simulink model "PI_model"  (Simulink 8.1)
settings: Solver=ode3  StartTime=0.0  StopTime=5500  FixedStep=1  RelTol=1e-3
undefined symbols (not defined in the file or in its folder): sys
libraries: simulink x2
settings Model: Creator=Lenovo  LastModifiedBy=Lenovo
settings DebuggingCC: FcnCallInpInsideContextMsg=EnableAllAsWarning

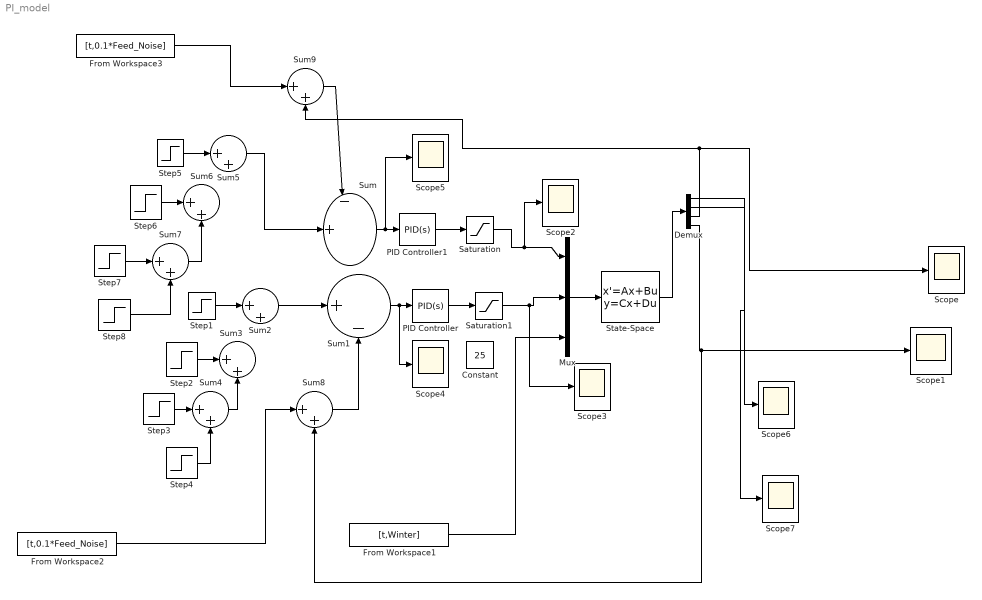
== system PI_model ==
  Constant : Constant  Value=25
  Demux : Demux
  From Workspace1 : FromWorkspace  VariableName=[t,Winter]  SampleTime=0
  From Workspace2 : FromWorkspace  VariableName=[t,0.1*Feed_Noise]  SampleTime=0
  From Workspace3 : FromWorkspace  VariableName=[t,0.1*Feed_Noise]  SampleTime=0
  Mux : Mux  Inputs=3
  PID Controller : simulink/Continuous/PID Controller  Controller=PID  TimeDomain=Continuous-time  SampleTime=1  IntegratorMethod=Forward Euler  FilterMethod=Forward Euler  Form=Parallel  P=8.594*0.5  I=0.17188*2  D=0  N=100  InitialConditionSource=internal  InitialConditionForIntegrator=0  InitialConditionForFilter=0  ExternalReset=none  LimitOutput=off  UpperSaturationLimit=inf  LowerSaturationLimit=-inf  LinearizeAsGain=off  AntiWindupMode=none  Kb=1  TrackingMode=off  Kt=1  PParamMin=[]  PParamMax=[]  IParamMin=[]  IParamMax=[]  DParamMin=[]  DParamMax=[]  NParamMin=[]  NParamMax=[]  KbParamMin=[]  KbParamMax=[]  KtParamMin=[]  KtParamMax=[]  POutMin=[]  POutMax=[]  IOutMin=[]  IOutMax=[]  DOutMin=[]  DOutMax=[]  NOutMin=[]  NOutMax=[]  KbOutMin=[]  KbOutMax=[]  KtOutMin=[]  KtOutMax=[]  IntegratorOutMin=[]  IntegratorOutMax=[]  FilterOutMin=[]  FilterOutMax=[]  SumOutMin=[]  SumOutMax=[]  SumI1OutMin=[]  SumI1OutMax=[]  SumI2OutMin=[]  SumI2OutMax=[]  SumI3OutMin=[]  SumI3OutMax=[]  SumDOutMin=[]  SumDOutMax=[]  SaturationOutMin=[]  SaturationOutMax=[]  IntegratorContinuousStateAttributes=''  IntegratorStateMustResolveToSignalObject=off  IntegratorRTWStateStorageClass=Auto  FilterContinuousStateAttributes=''  FilterStateMustResolveToSignalObject=off  FilterRTWStateStorageClass=Auto
  PID Controller1 : simulink/Continuous/PID Controller  Controller=PID  TimeDomain=Continuous-time  SampleTime=1  IntegratorMethod=Forward Euler  FilterMethod=Forward Euler  Form=Parallel  P=8.594*0.4  I=0.17188*5  D=0  N=100  InitialConditionSource=internal  InitialConditionForIntegrator=0  InitialConditionForFilter=0  ExternalReset=none  LimitOutput=off  UpperSaturationLimit=inf  LowerSaturationLimit=-inf  LinearizeAsGain=off  AntiWindupMode=none  Kb=1  TrackingMode=off  Kt=1  PParamMin=[]  PParamMax=[]  IParamMin=[]  IParamMax=[]  DParamMin=[]  DParamMax=[]  NParamMin=[]  NParamMax=[]  KbParamMin=[]  KbParamMax=[]  KtParamMin=[]  KtParamMax=[]  POutMin=[]  POutMax=[]  IOutMin=[]  IOutMax=[]  DOutMin=[]  DOutMax=[]  NOutMin=[]  NOutMax=[]  KbOutMin=[]  KbOutMax=[]  KtOutMin=[]  KtOutMax=[]  IntegratorOutMin=[]  IntegratorOutMax=[]  FilterOutMin=[]  FilterOutMax=[]  SumOutMin=[]  SumOutMax=[]  SumI1OutMin=[]  SumI1OutMax=[]  SumI2OutMin=[]  SumI2OutMax=[]  SumI3OutMin=[]  SumI3OutMax=[]  SumDOutMin=[]  SumDOutMax=[]  SaturationOutMin=[]  SaturationOutMax=[]  IntegratorContinuousStateAttributes=''  IntegratorStateMustResolveToSignalObject=off  IntegratorRTWStateStorageClass=Auto  FilterContinuousStateAttributes=''  FilterStateMustResolveToSignalObject=off  FilterRTWStateStorageClass=Auto
  Saturation : Saturate  UpperLimit=50  LowerLimit=15
  Saturation1 : Saturate  UpperLimit=50  LowerLimit=15
  Scope{,1..7} (8 alike) : Scope
      Scope settings: SaveName=NBT  MaxDataPoints=5500
      Scope1 settings: SaveName=SBT  MaxDataPoints=5500
      Scope2 settings: SaveName=swn_pi  MaxDataPoints=5500
      Scope3 settings: SaveName=sws_pi  MaxDataPoints=5500
      Scope4 settings: SaveName=ScopeData4
      Scope5 settings: SaveName=ScopeData5
      Scope6 settings: SaveName=RWN_pi  MaxDataPoints=5500
      Scope7 settings: SaveName=RWS_pi  MaxDataPoints=5500
  State-Space : StateSpace  A=sys.a  B=sys.b  C=sys.c  D=sys.d  X0=[26 28 23 23.5]  ContinuousStateAttributes='Temperature'
  Step1 : Step  Time=2000  Before=20  After=25  SampleTime=0
  Step2 : Step  Time=2000  After=-3  SampleTime=0
  Step3 : Step  Time=3000  After=4  SampleTime=0
  Step4 : Step  Time=4000  After=-3  SampleTime=0
  Step5 : Step  Time=2000  Before=20  After=25  SampleTime=0
  Step6 : Step  Time=2000  After=-3  SampleTime=0
  Step7 : Step  Time=3000  After=4  SampleTime=0
  Step8 : Step  Time=4000  After=-3  SampleTime=0
  Sum : Sum  Inputs=|-||||+||||||
  Sum1 : Sum  Inputs=|+-
  Sum{2..9} (8 alike) : Sum  Inputs=|++
  wires:
  State-Space/1 -> Demux/1
  Sum1/1 -> Scope4/1, PID Controller/1
  Sum/1 -> Scope5/1, PID Controller1/1
  Mux/1 -> State-Space/1
  Sum2/1 -> Sum1/1
  Step1/1 -> Sum2/1
  Step2/1 -> Sum3/1
  Sum4/1 -> Sum3/2
  Step3/1 -> Sum4/1
  Step4/1 -> Sum4/2
  Sum5/1 -> Sum/2
  Step5/1 -> Sum5/1
  Step6/1 -> Sum6/1
  Sum7/1 -> Sum6/2
  Step7/1 -> Sum7/1
  Step8/1 -> Sum7/2
  Demux/2 -> Scope7/1
  Demux/3 -> Scope/1, Sum9/2
  Demux/1 -> Scope6/1
  PID Controller1/1 -> Saturation/1
  Saturation/1 -> Mux/1, Scope2/1
  PID Controller/1 -> Saturation1/1
  Saturation1/1 -> Mux/2, Scope3/1
  From Workspace1/1 -> Mux/3
  Demux/4 -> Sum8/2, Scope1/1
  Sum8/1 -> Sum1/2
  From Workspace2/1 -> Sum8/1
  From Workspace3/1 -> Sum9/1
  Sum9/1 -> Sum/1
